simulink model "Controllo_assey_Rigido"  (R2021a)
settings: Solver=VariableStepAuto  StartTime=0.0  StopTime=5  RelTol=1e-3
values from neighbouring files (symbols this model uses):
  pary = parametriy ()    [mainy.m]
undefined symbols (not defined in the file or in its folder): Evaluate_Trajectory, m
libraries: cstblocks x2
settings Model: Creator=stefa  LastModifiedBy=stefa
settings DebuggingCC: AlgebraicLoopMsg=none

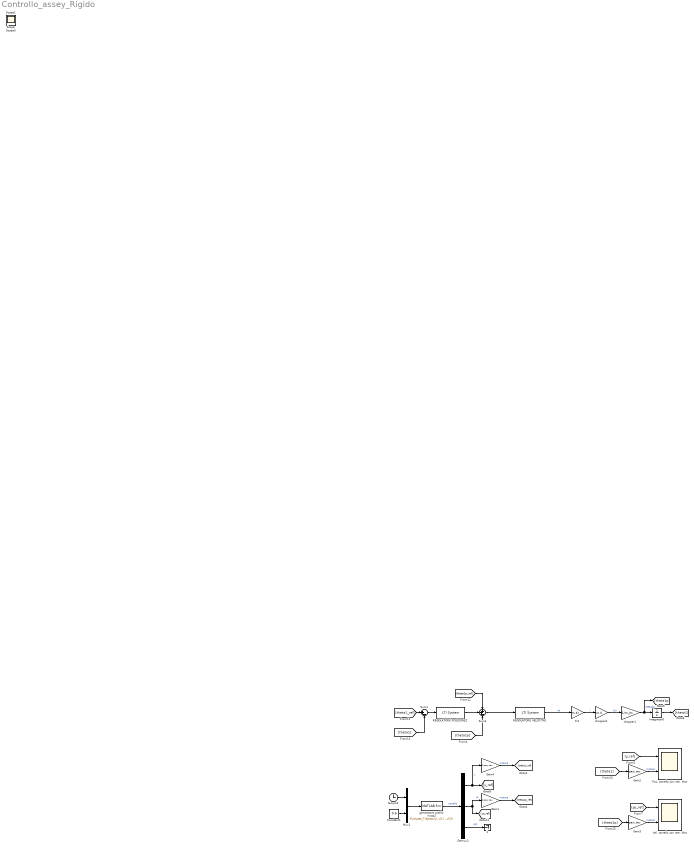
== system Controllo_assey_Rigido ==
  " 1" : Terminator
  Constant1 : Constant  Value=0.6
  Demux2 : Demux  Outputs=3
  Gain1 : Gain  Gain=1/pary.tau
  Gain2 : Gain  Gain=pary.tau
  Gain3 : Gain  Gain=pary.tau
  Gain4 : Gain  Gain=1/pary.tau
  Integrator6 : Integrator
  Kr1 : Gain  Gain=m.Kr
  Mux1 : Mux  Inputs=2
  Pos. carrello con retr. Mot : Scope  NumInputPorts=2
  REGOLATORE POSIZIONE2 : cstblocks/LTI System  sys=ap.H_P  IC=[]
  REGOLATORE VELOCITA1 : cstblocks/LTI System  sys=av.PI_V  IC=[]
  Sum1 : Sum  Inputs=|+-
  Sum4 : Sum  Inputs=++-
  Vel. carrello con retr. Mot : Scope  NumInputPorts=2
  chopper1 : Gain  Gain=1/m.Jm
  chopper2 : Gain  Gain=m.K
  generatore profilo moto2 : MATLABFcn  MATLABFcn=Evaluate_Trajectory( u(1) , u(2))  OutputDimensions=3
  tempo2 : Clock
  Scope : Scope
  Scope1 : Scope
  Scope3 : Scope
  wires:
  Demux2/3 -> " 1"/1  "YPP"
  Mux1/1 -> generatore profilo moto2/1
  generatore profilo moto2/1 -> Demux2/1  "carrello"
  Constant1/1 -> Mux1/2
  tempo2/1 -> Mux1/1
  Demux2/1 -> [y_ref], Gain4/1  "Y"
  Demux2/2 -> Gain1/1, [yp_ref]  "YP"
  Kr1/1 -> chopper2/1  "I"
  Sum1/1 -> REGOLATORE POSIZIONE2/1
  REGOLATORE POSIZIONE2/1 -> Sum4/2
  REGOLATORE VELOCITA1/1 -> Kr1/1  "Va"
  Sum4/1 -> REGOLATORE VELOCITA1/1
  [theta1p_ref] -> Sum4/1
  Gain4/1 -> [theta1_ref]  "motore"
  [theta1_ref] -> Sum1/1
  Gain1/1 -> [theta1p_ref]  "motore"
  [theta1p] -> Sum4/3
  [theta1] -> Sum1/2
  chopper1/1 -> [theta1p], Integrator6/1  "theta1p"
  Integrator6/1 -> [theta1]
  chopper2/1 -> chopper1/1  "Cm"
  [theta1] -> Gain2/1
  Gain2/1 -> Pos. carrello con retr. Mot/2  "motore"
  Gain3/1 -> Vel. carrello con retr. Mot/2  "motore"
  [y_ref] -> Pos. carrello con retr. Mot/1
  [yp_ref] -> Vel. carrello con retr. Mot/1
  [theta1p] -> Gain3/1
